simulink model "backups"  (R2024a)
settings: Solver=VariableStepAuto  StartTime=0.0  StopTime=10.0  RelTol=1e-3
values from neighbouring files (symbols this model uses):
  AttKd_x = inp(4,2).Var2    [SFF_Simulator_Entradas.m]
  AttKd_y = inp(5,2).Var2    [SFF_Simulator_Entradas.m]
  AttKd_z = inp(6,2).Var2    [SFF_Simulator_Entradas.m]
  AttKp_x = inp(1,2).Var2    [SFF_Simulator_Entradas.m]
  AttKp_y = inp(2,2).Var2    [SFF_Simulator_Entradas.m]
  AttKp_z = inp(3,2).Var2    [SFF_Simulator_Entradas.m]
  B = inp(8,2).Var2    [SFF_Simulator_Entradas.m]
  beta = inp(2,2).Var2    [SFF_Simulator_Entradas.m]
  Cd1 = inp(4,2).Var2    [SFF_Simulator_Entradas.m]
  cdgps = inp(1,2).Var2    [SFF_Simulator_Entradas.m]
  estrelas = inp(4,2).Var2    [SFF_Simulator_Entradas.m]
  estrelas_bias = inp(6,2).Var2    [SFF_Simulator_Entradas.m]
  estrelas_ruido = inp(5,2).Var2    [SFF_Simulator_Entradas.m]
  Fn = inp(2,2).Var2    [SFF_Simulator_Entradas.m]
  gps_bias = inp(3,2).Var2    [SFF_Simulator_Entradas.m]
  gps_ruido = inp(2,2).Var2    [SFF_Simulator_Entradas.m]
  Iw = inp(7,2).Var2    [SFF_Simulator_Entradas.m]
  Ixx = inp(7,2).Var2    [SFF_Simulator_Entradas.m]
  Iyy = inp(8,2).Var2    [SFF_Simulator_Entradas.m]
  Izz = inp(9,2).Var2    [SFF_Simulator_Entradas.m]
  Km = inp(3,2).Var2    [SFF_Simulator_Entradas.m]
  Kv = inp(9,2).Var2    [SFF_Simulator_Entradas.m]
  L1 = inp(5,2).Var2    [SFF_Simulator_Entradas.m]
  limCorrente = inp(4,2).Var2    [SFF_Simulator_Entradas.m]
  limVolt = inp(5,2).Var2    [SFF_Simulator_Entradas.m]
  m1 = inp(6,2).Var2    [SFF_Simulator_Entradas.m]
  magne = inp(10,2).Var2    [SFF_Simulator_Entradas.m]
  magne_bias = inp(12,2).Var2    [SFF_Simulator_Entradas.m]
  magne_ruido = inp(11,2).Var2    [SFF_Simulator_Entradas.m]
  man = inp(1,2).Var2    [SFF_Simulator_Entradas.m]
  OrbKd_x = inp(3,2).Var2    [SFF_Simulator_Entradas.m]
  OrbKd_y = inp(6,2).Var2    [SFF_Simulator_Entradas.m]
  OrbKd_z = inp(9,2).Var2    [SFF_Simulator_Entradas.m]
  OrbKi_x = inp(2,2).Var2    [SFF_Simulator_Entradas.m]
  OrbKi_y = inp(5,2).Var2    [SFF_Simulator_Entradas.m]
  OrbKi_z = inp(8,2).Var2    [SFF_Simulator_Entradas.m]
  OrbKp_x = inp(1,2).Var2    [SFF_Simulator_Entradas.m]
  OrbKp_y = inp(4,2).Var2    [SFF_Simulator_Entradas.m]
  OrbKp_z = inp(7,2).Var2    [SFF_Simulator_Entradas.m]
  propForcaAtivo = inp(1,2).Var2    [SFF_Simulator_Entradas.m]
  Rm = inp(6,2).Var2    [SFF_Simulator_Entradas.m]
  rodaAtivo = inp(1,2).Var2    [SFF_Simulator_Entradas.m]
  RodKi = inp(1,2).Var2    [SFF_Simulator_Entradas.m]
  sat_torquerod = inp(14,2).Var2    [SFF_Simulator_Entradas.m]
  torqrodAtivo = inp(1,2).Var2    [SFF_Simulator_Entradas.m]
undefined symbols (not defined in the file or in its folder): IAU, J2, mi, omega_E, propMomentoAtivo, Re, sat_rodareacao, WMM2020
libraries: dspsrcs4 x19, aerolibtransform2 x2, aerolibgravity2 x2, simulink x1
(part 2 of 4)

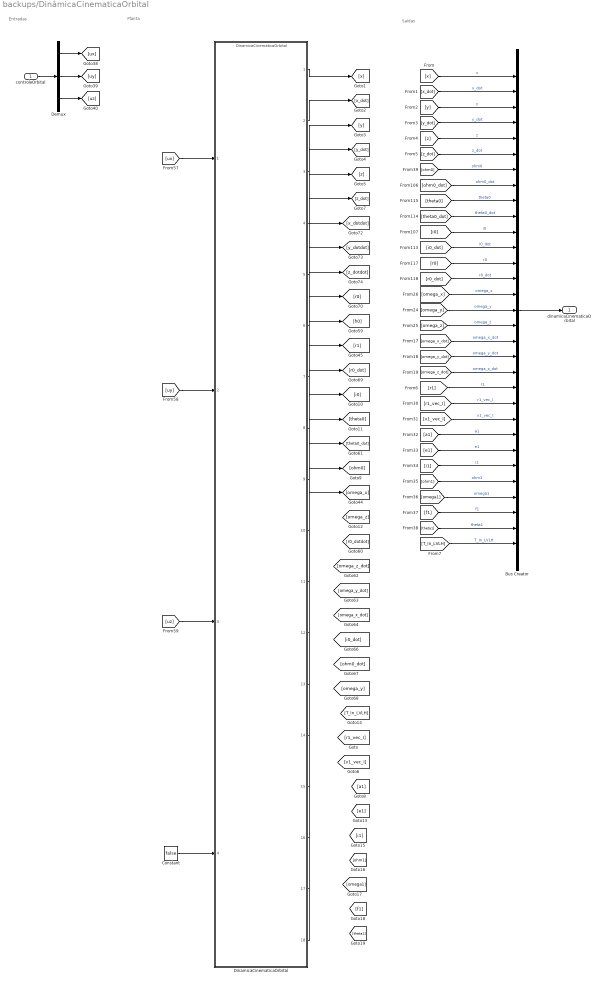
== system backups/DinâmicaCinematicaOrbital ==
  note: Entradas
  note: Saídas
  note: Planta
  controleOrbital : Inport  OutDataTypeStr=double
  Bus Creator : BusCreator  Inputs=31
  Constant : Constant  Value=false
  Demux : Demux  Outputs=3
  DinamicaCinematicaOrbital : ModelReference  ModelNameDialog=DinamicaCinematicaOrbital  ModelReferenceVersion=5.18
  dinamicaCinematicaOrbital : Outport
  wires:
  [x] -> Bus Creator/1  "x"
  [z_dot] -> Bus Creator/6  "z_dot"
  [y] -> Bus Creator/3  "y"
  [z] -> Bus Creator/5  "z"
  [x_dot] -> Bus Creator/2  "x_dot"
  [y_dot] -> Bus Creator/4  "y_dot"
  Bus Creator/1 -> dinamicaCinematicaOrbital/1
  controleOrbital/1 -> Demux/1
  Demux/1 -> [ux]
  Demux/2 -> [uy]
  Demux/3 -> [uz]
  [ohm0] -> Bus Creator/7  "ohm0"
  [ohm0_dot] -> Bus Creator/8  "ohm0_dot"
  [theta0] -> Bus Creator/9  "theta0"
  [theta0_dot] -> Bus Creator/10  "theta0_dot"
  [i0] -> Bus Creator/11  "i0"
  [i0_dot] -> Bus Creator/12  "i0_dot"
  [r0] -> Bus Creator/13  "r0"
  [r0_dot] -> Bus Creator/14  "r0_dot"
  [omega_x] -> Bus Creator/15  "omega_x"
  [omega_y] -> Bus Creator/16  "omega_y"
  [omega_z] -> Bus Creator/17  "omega_z"
  [omega_x_dot] -> Bus Creator/18  "omega_x_dot"
  [omega_y_dot] -> Bus Creator/19  "omega_y_dot"
  [omega_z_dot] -> Bus Creator/20  "omega_z_dot"
  [r1] -> Bus Creator/21  "r1"
  [r1_vec_I] -> Bus Creator/22  "r1_vec_I"
  [v1_vec_I] -> Bus Creator/23  "v1_vec_I"
  [a1] -> Bus Creator/24  "a1"
  [e1] -> Bus Creator/25  "e1"
  [i1] -> Bus Creator/26  "i1"
  [ohm1] -> Bus Creator/27  "ohm1"
  [omega1] -> Bus Creator/28  "omega1"
  [f1] -> Bus Creator/29  "f1"
  [theta1] -> Bus Creator/30  "theta1"
  [T_In_LVLH] -> Bus Creator/31  "T_In_LVLH"
  [ux] -> DinamicaCinematicaOrbital/1
  [uy] -> DinamicaCinematicaOrbital/2
  [uz] -> DinamicaCinematicaOrbital/3
  Constant/1 -> DinamicaCinematicaOrbital/4
  DinamicaCinematicaOrbital/7 -> [x_dotdot]
  DinamicaCinematicaOrbital/8 -> [y_dotdot]
  DinamicaCinematicaOrbital/9 -> [z_dotdot]
  DinamicaCinematicaOrbital/10 -> [r0]
  DinamicaCinematicaOrbital/11 -> [h0]
  DinamicaCinematicaOrbital/12 -> [r1]
  DinamicaCinematicaOrbital/13 -> [r0_dot]
  DinamicaCinematicaOrbital/14 -> [i0]
  DinamicaCinematicaOrbital/15 -> [theta0]
  DinamicaCinematicaOrbital/16 -> [theta0_dot]
  DinamicaCinematicaOrbital/17 -> [ohm0]
  DinamicaCinematicaOrbital/18 -> [omega_x]
  ? -> [omega_z]
  ? -> [r0_dotdot]
  ? -> [omega_z_dot]
  ? -> [omega_y_dot]
  ? -> [omega_x_dot]
  ? -> [i0_dot]
  ? -> [ohm0_dot]
  ? -> [omega_y]
  ? -> [T_In_LVLH]
  DinamicaCinematicaOrbital/1 -> [x]
  DinamicaCinematicaOrbital/2 -> [x_dot]
  DinamicaCinematicaOrbital/4 -> [y_dot]
  DinamicaCinematicaOrbital/5 -> [z]
  DinamicaCinematicaOrbital/6 -> [z_dot]
  DinamicaCinematicaOrbital/3 -> [y]
  ? -> [r1_vec_I]
  ? -> [v1_vec_I]
  ? -> [theta1]
  ? -> [f1]
  ? -> [omega1]
  ? -> [ohm1]
  ? -> [i1]
  ? -> [e1]
  ? -> [a1]

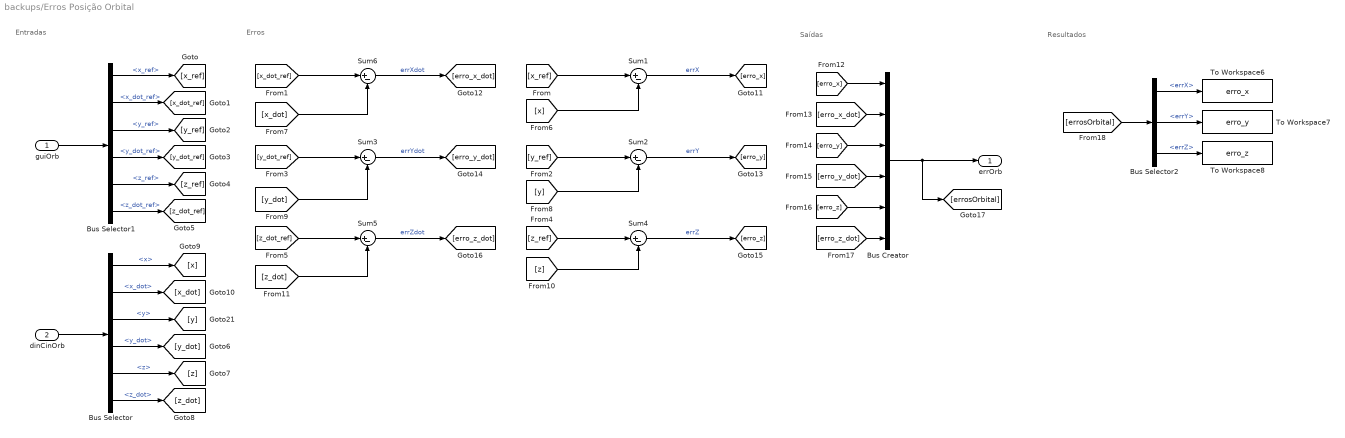
== system backups/Erros Posição Orbital ==
  note: Saídas
  note: Erros
  note: Entradas
  note: Resultados
  guiOrb : Inport
  dinCinOrb : Inport  Port=2
  Bus Creator : BusCreator  Inputs=6
  Bus Selector : BusSelector  OutputSignals=x,x_dot,y,y_dot,z,z_dot
  Bus Selector1 : BusSelector  OutputSignals=x_ref,x_dot_ref,y_ref,y_dot_ref,z_ref,z_dot_ref
  Bus Selector2 : BusSelector  OutputSignals=errX,errY,errZ
  Sum{1..6} (6 alike) : Sum  Inputs=|+-
  To Workspace6 : ToWorkspace  VariableName=erro_x  SampleTime=-1
      settings: Save2DSignal=2-D array (concatenate along first dimension)
  To Workspace7 : ToWorkspace  VariableName=erro_y  SampleTime=-1
      settings: Save2DSignal=2-D array (concatenate along first dimension)
  To Workspace8 : ToWorkspace  VariableName=erro_z  SampleTime=-1
      settings: Save2DSignal=2-D array (concatenate along first dimension)
  errOrb : Outport
  wires:
  [x] -> Sum1/2
  [x_dot] -> Sum6/2
  [x_dot_ref] -> Sum6/1
  [x_ref] -> Sum1/1
  Sum6/1 -> [erro_x_dot]  "errXdot"
  Sum1/1 -> [erro_x]  "errX"
  Sum3/1 -> [erro_y_dot]  "errYdot"
  Sum2/1 -> [erro_y]  "errY"
  [y] -> Sum2/2
  [y_dot] -> Sum3/2
  [y_ref] -> Sum2/1
  [y_dot_ref] -> Sum3/1
  Sum5/1 -> [erro_z_dot]  "errZdot"
  Sum4/1 -> [erro_z]  "errZ"
  [z_dot] -> Sum5/2
  [z_dot_ref] -> Sum5/1
  [z] -> Sum4/2
  [z_ref] -> Sum4/1
  Bus Selector1/4 -> [y_dot_ref]  "<y_dot_ref>"
  Bus Selector1/2 -> [x_dot_ref]  "<x_dot_ref>"
  guiOrb/1 -> Bus Selector1/1
  Bus Selector1/6 -> [z_dot_ref]  "<z_dot_ref>"
  Bus Selector1/3 -> [y_ref]  "<y_ref>"
  Bus Selector1/1 -> [x_ref]  "<x_ref>"
  Bus Selector1/5 -> [z_ref]  "<z_ref>"
  Bus Selector/1 -> [x]  "<x>"
  Bus Selector/4 -> [y_dot]  "<y_dot>"
  Bus Selector/3 -> [y]  "<y>"
  Bus Selector/6 -> [z_dot]  "<z_dot>"
  Bus Selector/5 -> [z]  "<z>"
  Bus Selector/2 -> [x_dot]  "<x_dot>"
  dinCinOrb/1 -> Bus Selector/1
  [erro_x] -> Bus Creator/1
  [erro_x_dot] -> Bus Creator/2
  [erro_y] -> Bus Creator/3
  [erro_y_dot] -> Bus Creator/4
  [erro_z] -> Bus Creator/5
  [erro_z_dot] -> Bus Creator/6
  Bus Selector2/2 -> To Workspace7/1  "<errY>"
  Bus Selector2/3 -> To Workspace8/1  "<errZ>"
  Bus Selector2/1 -> To Workspace6/1  "<errX>"
  [errosOrbital] -> Bus Selector2/1
  Bus Creator/1 -> [errosOrbital], errOrb/1

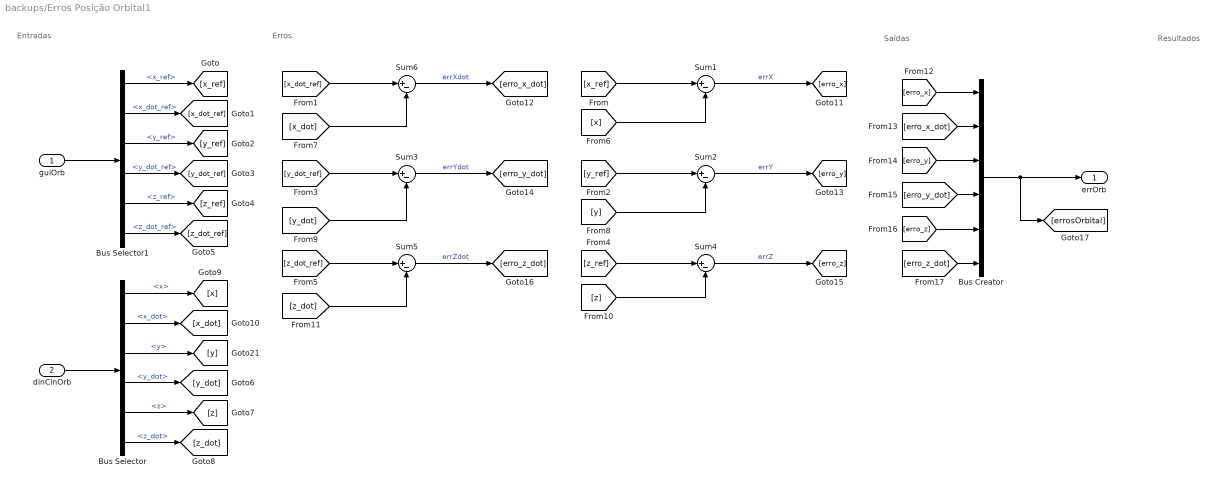
== system backups/Erros Posição Orbital1 ==
  note: Saídas
  note: Erros
  note: Entradas
  note: Resultados
  guiOrb : Inport
  dinCinOrb : Inport  Port=2
  Bus Creator : BusCreator  Inputs=6
  Bus Selector : BusSelector  OutputSignals=x,x_dot,y,y_dot,z,z_dot
  Bus Selector1 : BusSelector  OutputSignals=x_ref,x_dot_ref,y_ref,y_dot_ref,z_ref,z_dot_ref
  Sum{1..6} (6 alike) : Sum  Inputs=|+-
  errOrb : Outport
  wires:
  [x] -> Sum1/2
  [x_dot] -> Sum6/2
  [x_dot_ref] -> Sum6/1
  [x_ref] -> Sum1/1
  Sum6/1 -> [erro_x_dot]  "errXdot"
  Sum1/1 -> [erro_x]  "errX"
  Sum3/1 -> [erro_y_dot]  "errYdot"
  Sum2/1 -> [erro_y]  "errY"
  [y] -> Sum2/2
  [y_dot] -> Sum3/2
  [y_ref] -> Sum2/1
  [y_dot_ref] -> Sum3/1
  Sum5/1 -> [erro_z_dot]  "errZdot"
  Sum4/1 -> [erro_z]  "errZ"
  [z_dot] -> Sum5/2
  [z_dot_ref] -> Sum5/1
  [z] -> Sum4/2
  [z_ref] -> Sum4/1
  Bus Selector1/4 -> [y_dot_ref]  "<y_dot_ref>"
  Bus Selector1/2 -> [x_dot_ref]  "<x_dot_ref>"
  guiOrb/1 -> Bus Selector1/1
  Bus Selector1/6 -> [z_dot_ref]  "<z_dot_ref>"
  Bus Selector1/3 -> [y_ref]  "<y_ref>"
  Bus Selector1/1 -> [x_ref]  "<x_ref>"
  Bus Selector1/5 -> [z_ref]  "<z_ref>"
  Bus Selector/1 -> [x]  "<x>"
  Bus Selector/4 -> [y_dot]  "<y_dot>"
  Bus Selector/3 -> [y]  "<y>"
  Bus Selector/6 -> [z_dot]  "<z_dot>"
  Bus Selector/5 -> [z]  "<z>"
  Bus Selector/2 -> [x_dot]  "<x_dot>"
  dinCinOrb/1 -> Bus Selector/1
  [erro_x] -> Bus Creator/1
  [erro_x_dot] -> Bus Creator/2
  [erro_y] -> Bus Creator/3
  [erro_y_dot] -> Bus Creator/4
  [erro_z] -> Bus Creator/5
  [erro_z_dot] -> Bus Creator/6
  Bus Creator/1 -> [errosOrbital], errOrb/1

== system backups/Erros Quatérnions ==
  note: Erros
  note: Saídas
  note: Entradas
  q_ref : Inport
  q_rel : Inport  Port=2
  MATLAB Function4 : MATLAB Function  TreatAsAtomicUnit=on
  q_erro : Outport
  wires:
  [q_ref] -> MATLAB Function4/1(q_d)
  [q_rel] -> MATLAB Function4/2(q)
  MATLAB Function4/1(q_error) -> [q_erro]  "q_erro"
  [q_erro] -> q_erro/1
  q_rel/1 -> [q_rel]
  q_ref/1 -> [q_ref]

== system backups/Erros Quatérnions1 ==
  note: Erros
  note: Saídas
  note: Entradas
  q_ref : Inport
  q_rel : Inport  Port=2
  MATLAB Function4 : MATLAB Function  TreatAsAtomicUnit=on
  Scope : Scope
  q_erro : Outport
  wires:
  [q_ref] -> MATLAB Function4/1(q_d)
  [q_rel] -> MATLAB Function4/2(q)
  MATLAB Function4/1(q_error) -> [q_erro]  "q_erro"
  [q_erro] -> Scope/1, q_erro/1
  q_rel/1 -> [q_rel]
  q_ref/1 -> [q_ref]

== system backups/Guiamento Atitude ==
  note: Entradas
  note: Guiamento de Atitude
  note: Saídas
  note: Resultados
  dinCinOrb : Inport
  Bus Selector1 : BusSelector  OutputSignals=T_In_LVLH,r0,ohm1,i1,theta1,r1_vec_I
  "Euler -> Quatérnions" : MATLAB Function  TreatAsAtomicUnit=on
  GuiamentoAtitude : ModelReference  ModelNameDialog=GuiamentoAtitude  ModelReferenceVersion=3.9
  To Workspace12 : ToWorkspace  VariableName=phi_ref  SampleTime=-1
      settings: Save2DSignal=2-D array (concatenate along first dimension)
  To Workspace13 : ToWorkspace  VariableName=theta_ref  SampleTime=-1
      settings: Save2DSignal=2-D array (concatenate along first dimension)
  To Workspace14 : ToWorkspace  VariableName=psi_ref  SampleTime=-1
      settings: Save2DSignal=2-D array (concatenate along first dimension)
  q_ref : Outport
  wires:
  dinCinOrb/1 -> Bus Selector1/1
  GuiamentoAtitude/2 -> [theta_ref]
  [r0] -> GuiamentoAtitude/2
  [ohm1] -> GuiamentoAtitude/3
  [theta1] -> GuiamentoAtitude/5
  GuiamentoAtitude/1 -> [phi_ref]
  GuiamentoAtitude/3 -> [psi_ref]
  [r1_vec_I] -> GuiamentoAtitude/6
  [i1] -> GuiamentoAtitude/4
  [T_In_LVLH] -> GuiamentoAtitude/1
  [theta_ref] -> To Workspace13/1
  [phi_ref] -> To Workspace12/1
  [phi_ref] -> "Euler -> Quatérnions"/1(phi_ref)
  [psi_ref] -> "Euler -> Quatérnions"/3(psi_ref)
  [psi_ref] -> To Workspace14/1
  [theta_ref] -> "Euler -> Quatérnions"/2(theta_ref)
  "Euler -> Quatérnions"/1(q_ref) -> q_ref/1
  Bus Selector1/3 -> [ohm1]  "<ohm1>"
  Bus Selector1/5 -> [theta1]  "<theta1>"
  Bus Selector1/2 -> [r0]  "<r0>"
  Bus Selector1/4 -> [i1]  "<i1>"
  Bus Selector1/1 -> [T_In_LVLH]  "<T_In_LVLH>"
  Bus Selector1/6 -> [r1_vec_I]  "<r1_vec_I>"

== system backups/Guiamento Atitude1 ==
  note: Entradas
  note: Guiamento de Atitude
  note: Saídas
  note: Resultados
  dinCinOrb : Inport
  Bus Selector1 : BusSelector  OutputSignals=T_In_LVLH,r0,ohm1,i1,theta1,r1_vec_I
  "Euler -> Quatérnions" : MATLAB Function  TreatAsAtomicUnit=on
  GuiamentoAtitude : ModelReference  ModelNameDialog=GuiamentoAtitude  ModelReferenceVersion=3.9
  To Workspace12 : ToWorkspace  VariableName=phi_ref  SampleTime=-1
      settings: Save2DSignal=2-D array (concatenate along first dimension)
  To Workspace13 : ToWorkspace  VariableName=theta_ref  SampleTime=-1
      settings: Save2DSignal=2-D array (concatenate along first dimension)
  To Workspace14 : ToWorkspace  VariableName=psi_ref  SampleTime=-1
      settings: Save2DSignal=2-D array (concatenate along first dimension)
  q_ref : Outport
  wires:
  dinCinOrb/1 -> Bus Selector1/1
  GuiamentoAtitude/2 -> [theta_ref]
  [r0] -> GuiamentoAtitude/2
  [ohm1] -> GuiamentoAtitude/3
  [theta1] -> GuiamentoAtitude/5
  GuiamentoAtitude/1 -> [phi_ref]
  GuiamentoAtitude/3 -> [psi_ref]
  [r1_vec_I] -> GuiamentoAtitude/6
  [i1] -> GuiamentoAtitude/4
  [T_In_LVLH] -> GuiamentoAtitude/1
  [theta_ref] -> To Workspace13/1
  [phi_ref] -> To Workspace12/1
  [phi_ref] -> "Euler -> Quatérnions"/1(phi_ref)
  [psi_ref] -> "Euler -> Quatérnions"/3(psi_ref)
  [psi_ref] -> To Workspace14/1
  [theta_ref] -> "Euler -> Quatérnions"/2(theta_ref)
  "Euler -> Quatérnions"/1(q_ref) -> q_ref/1
  Bus Selector1/3 -> [ohm1]  "<ohm1>"
  Bus Selector1/5 -> [theta1]  "<theta1>"
  Bus Selector1/2 -> [r0]  "<r0>"
  Bus Selector1/4 -> [i1]  "<i1>"
  Bus Selector1/1 -> [T_In_LVLH]  "<T_In_LVLH>"
  Bus Selector1/6 -> [r1_vec_I]  "<r1_vec_I>"

== system backups/Guiamento Orbital ==
  note: Saídas
  note: Guiamento Orbital
  note: Resultados
  Bus Creator : BusCreator  Inputs=12
  Bus Selector : BusSelector  OutputSignals=x_ref,y_ref,z_ref
  Constant13 : Constant  Value=man  OutDataTypeStr=boolean
  DinamicaCinematicaOrbital : ModelReference  ModelNameDialog=DinamicaCinematicaOrbital  ModelReferenceVersion=5.18
  Terminator{,1..5} (6 alike) : Terminator
  To Workspace : ToWorkspace  VariableName=x_ref  SampleTime=-1
      settings: Save2DSignal=2-D array (concatenate along first dimension)
  To Workspace1 : ToWorkspace  VariableName=y_ref  SampleTime=-1
      settings: Save2DSignal=2-D array (concatenate along first dimension)
  To Workspace2 : ToWorkspace  VariableName=z_ref  SampleTime=-1
      settings: Save2DSignal=2-D array (concatenate along first dimension)
  ux : Constant  Value=0
  uy : Constant  Value=0
  uz : Constant  Value=0
  guiOrb : Outport
  wires:
  [x] -> Bus Creator/1  "x_ref"
  [x_dot] -> Bus Creator/2  "x_dot_ref"
  [y] -> Bus Creator/3  "y_ref"
  [y_dot] -> Bus Creator/4  "y_dot_ref"
  [z] -> Bus Creator/5  "z_ref"
  [z_dot] -> Bus Creator/6  "z_dot_ref"
  Bus Creator/1 -> [guiOrb], guiOrb/1
  ux/1 -> DinamicaCinematicaOrbital/1
  uy/1 -> DinamicaCinematicaOrbital/2
  uz/1 -> DinamicaCinematicaOrbital/3
  Constant13/1 -> DinamicaCinematicaOrbital/4
  [r0] -> Bus Creator/8  "r0"
  [T_In_LVLH] -> Bus Creator/7  "T_In_LVLH"
  [ohm1] -> Bus Creator/9  "ohm1"
  [i1] -> Bus Creator/10  "i1"
  [theta1] -> Bus Creator/11  "theta1"
  [r1_vec_I] -> Bus Creator/12  "r1_vec_I"
  Bus Selector/3 -> To Workspace2/1  "<z_ref>"
  Bus Selector/2 -> To Workspace1/1  "<y_ref>"
  Bus Selector/1 -> To Workspace/1  "<x_ref>"
  [guiOrb] -> Bus Selector/1
  DinamicaCinematicaOrbital/1 -> [x]
  DinamicaCinematicaOrbital/2 -> [x_dot]
  DinamicaCinematicaOrbital/3 -> [y]
  DinamicaCinematicaOrbital/4 -> [y_dot]
  DinamicaCinematicaOrbital/5 -> [z]
  DinamicaCinematicaOrbital/6 -> [z_dot]
  DinamicaCinematicaOrbital/7 -> [r0]
  DinamicaCinematicaOrbital/8 -> Terminator/1
  DinamicaCinematicaOrbital/9 -> Terminator1/1
  DinamicaCinematicaOrbital/10 -> Terminator2/1
  DinamicaCinematicaOrbital/11 -> Terminator4/1
  DinamicaCinematicaOrbital/12 -> Terminator5/1
  DinamicaCinematicaOrbital/18 -> [theta1]
  DinamicaCinematicaOrbital/17 -> [ohm1]
  DinamicaCinematicaOrbital/16 -> [i1]
  DinamicaCinematicaOrbital/15 -> [r1_vec_I]
  DinamicaCinematicaOrbital/14 -> [T_In_LVLH]
  DinamicaCinematicaOrbital/13 -> Terminator3/1

== system backups/Guiamento Orbital1 ==
  note: Saídas
  note: Guiamento Orbital
  note: Resultados
  Bus Creator : BusCreator  Inputs=12
  Bus Selector : BusSelector  OutputSignals=x_ref,y_ref,z_ref
  Constant13 : Constant  Value=man  OutDataTypeStr=boolean
  DinamicaCinematicaOrbital : ModelReference  ModelNameDialog=DinamicaCinematicaOrbital  ModelReferenceVersion=5.18
  Terminator{,1..5} (6 alike) : Terminator
  To Workspace : ToWorkspace  VariableName=x_ref  SampleTime=-1
      settings: Save2DSignal=2-D array (concatenate along first dimension)
  To Workspace1 : ToWorkspace  VariableName=y_ref  SampleTime=-1
      settings: Save2DSignal=2-D array (concatenate along first dimension)
  To Workspace2 : ToWorkspace  VariableName=z_ref  SampleTime=-1
      settings: Save2DSignal=2-D array (concatenate along first dimension)
  ux : Constant  Value=0
  uy : Constant  Value=0
  uz : Constant  Value=0
  guiOrb : Outport
  wires:
  [x] -> Bus Creator/1  "x_ref"
  [x_dot] -> Bus Creator/2  "x_dot_ref"
  [y] -> Bus Creator/3  "y_ref"
  [y_dot] -> Bus Creator/4  "y_dot_ref"
  [z] -> Bus Creator/5  "z_ref"
  [z_dot] -> Bus Creator/6  "z_dot_ref"
  Bus Creator/1 -> [guiOrb], guiOrb/1
  ux/1 -> DinamicaCinematicaOrbital/1
  uy/1 -> DinamicaCinematicaOrbital/2
  uz/1 -> DinamicaCinematicaOrbital/3
  Constant13/1 -> DinamicaCinematicaOrbital/4
  [r0] -> Bus Creator/8  "r0"
  [T_In_LVLH] -> Bus Creator/7  "T_In_LVLH"
  [ohm1] -> Bus Creator/9  "ohm1"
  [i1] -> Bus Creator/10  "i1"
  [theta1] -> Bus Creator/11  "theta1"
  [r1_vec_I] -> Bus Creator/12  "r1_vec_I"
  Bus Selector/3 -> To Workspace2/1  "<z_ref>"
  Bus Selector/2 -> To Workspace1/1  "<y_ref>"
  Bus Selector/1 -> To Workspace/1  "<x_ref>"
  [guiOrb] -> Bus Selector/1
  DinamicaCinematicaOrbital/1 -> [x]
  DinamicaCinematicaOrbital/2 -> [x_dot]
  DinamicaCinematicaOrbital/3 -> [y]
  DinamicaCinematicaOrbital/4 -> [y_dot]
  DinamicaCinematicaOrbital/5 -> [z]
  DinamicaCinematicaOrbital/6 -> [z_dot]
  DinamicaCinematicaOrbital/7 -> [r0]
  DinamicaCinematicaOrbital/8 -> Terminator/1
  DinamicaCinematicaOrbital/9 -> Terminator1/1
  DinamicaCinematicaOrbital/10 -> Terminator2/1
  DinamicaCinematicaOrbital/11 -> Terminator4/1
  DinamicaCinematicaOrbital/12 -> Terminator5/1
  DinamicaCinematicaOrbital/18 -> [theta1]
  DinamicaCinematicaOrbital/17 -> [ohm1]
  DinamicaCinematicaOrbital/16 -> [i1]
  DinamicaCinematicaOrbital/15 -> [r1_vec_I]
  DinamicaCinematicaOrbital/14 -> [T_In_LVLH]
  DinamicaCinematicaOrbital/13 -> Terminator3/1

== system backups/GuiamentoAtitude ==
  note: Entradas
  note: Planta
  note: Saídas
  dinamicaCinematicaOrbital : Inport
  Bus Creator : BusCreator  Inputs=3
  Bus Selector : BusSelector  OutputSignals=T_In_LVLH,r0,ohm1,i1,theta1,r1_vec_I
  "Euler -> Quatérnions" : MATLAB Function  TreatAsAtomicUnit=on
  GuiamentoAtitude1 : ModelReference  ModelNameDialog=GuiamentoAtitude  ModelReferenceVersion=3.9
  eulerRef : Outport
  q_ref : Outport  Port=2
  wires:
  dinamicaCinematicaOrbital/1 -> Bus Selector/1
  Bus Selector/1 -> [T_In_LVLH]  "<T_In_LVLH>"
  Bus Selector/2 -> [r0]  "<r0>"
  Bus Selector/3 -> [ohm1]  "<ohm1>"
  Bus Selector/4 -> [i1]  "<i1>"
  Bus Selector/5 -> [theta1]  "<theta1>"
  Bus Selector/6 -> [r1_vec_I]  "<r1_vec_I>"
  GuiamentoAtitude1/2 -> [theta_ref]
  [r0] -> GuiamentoAtitude1/2
  [ohm1] -> GuiamentoAtitude1/3
  [theta1] -> GuiamentoAtitude1/5
  GuiamentoAtitude1/1 -> [phi_ref]
  GuiamentoAtitude1/3 -> [psi_ref]
  [r1_vec_I] -> GuiamentoAtitude1/6
  [i1] -> GuiamentoAtitude1/4
  [T_In_LVLH] -> GuiamentoAtitude1/1
  Bus Creator/1 -> eulerRef/1
  [theta_ref] -> Bus Creator/2  "theta_ref"
  [phi_ref] -> Bus Creator/1  "phi_ref"
  [phi_ref] -> "Euler -> Quatérnions"/1(phi_ref)
  [psi_ref] -> "Euler -> Quatérnions"/3(psi_ref)
  [psi_ref] -> Bus Creator/3  "psi_ref"
  [theta_ref] -> "Euler -> Quatérnions"/2(theta_ref)
  "Euler -> Quatérnions"/1(q_ref) -> q_ref/1

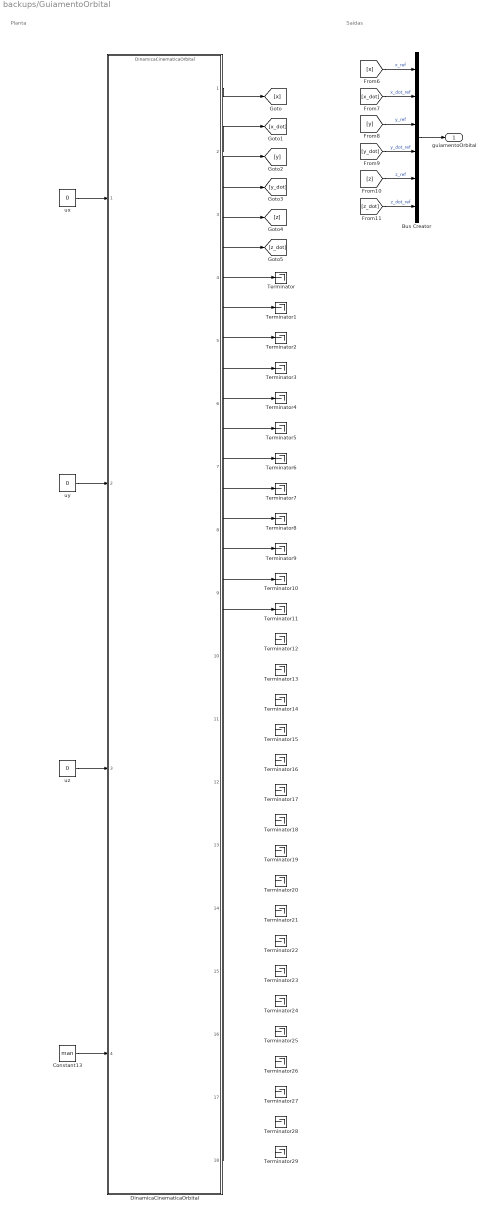
== system backups/GuiamentoOrbital ==
  note: Saídas
  note: Planta
  Bus Creator : BusCreator  Inputs=6
  Constant13 : Constant  Value=man  OutDataTypeStr=boolean
  DinamicaCinematicaOrbital : ModelReference  ModelNameDialog=DinamicaCinematicaOrbital  ModelReferenceVersion=5.18
  Terminator{,1..29} (30 alike) : Terminator
  ux : Constant  Value=0
  uy : Constant  Value=0
  uz : Constant  Value=0
  guiamentoOrbital : Outport
  wires:
  [x] -> Bus Creator/1  "x_ref"
  [x_dot] -> Bus Creator/2  "x_dot_ref"
  [y] -> Bus Creator/3  "y_ref"
  [y_dot] -> Bus Creator/4  "y_dot_ref"
  [z] -> Bus Creator/5  "z_ref"
  [z_dot] -> Bus Creator/6  "z_dot_ref"
  Bus Creator/1 -> guiamentoOrbital/1
  ux/1 -> DinamicaCinematicaOrbital/1
  uy/1 -> DinamicaCinematicaOrbital/2
  uz/1 -> DinamicaCinematicaOrbital/3
  DinamicaCinematicaOrbital/1 -> [x]
  DinamicaCinematicaOrbital/2 -> [x_dot]
  DinamicaCinematicaOrbital/3 -> [y]
  DinamicaCinematicaOrbital/4 -> [y_dot]
  DinamicaCinematicaOrbital/5 -> [z]
  DinamicaCinematicaOrbital/6 -> [z_dot]
  DinamicaCinematicaOrbital/7 -> Terminator/1
  DinamicaCinematicaOrbital/8 -> Terminator1/1
  DinamicaCinematicaOrbital/9 -> Terminator2/1
  DinamicaCinematicaOrbital/10 -> Terminator3/1
  DinamicaCinematicaOrbital/11 -> Terminator4/1
  DinamicaCinematicaOrbital/12 -> Terminator5/1
  DinamicaCinematicaOrbital/13 -> Terminator6/1
  DinamicaCinematicaOrbital/14 -> Terminator7/1
  DinamicaCinematicaOrbital/15 -> Terminator8/1
  DinamicaCinematicaOrbital/16 -> Terminator9/1
  DinamicaCinematicaOrbital/17 -> Terminator10/1
  DinamicaCinematicaOrbital/18 -> Terminator11/1
  ? -> Terminator12/1
  ? -> Terminator13/1
  ? -> Terminator14/1
  ? -> Terminator15/1
  ? -> Terminator16/1
  ? -> Terminator17/1
  ? -> Terminator18/1
  ? -> Terminator19/1
  Constant13/1 -> DinamicaCinematicaOrbital/4
  ? -> Terminator20/1
  ? -> Terminator21/1
  ? -> Terminator22/1
  ? -> Terminator23/1
  ? -> Terminator24/1
  ? -> Terminator25/1
  ? -> Terminator26/1
  ? -> Terminator27/1
  ? -> Terminator28/1
  ? -> Terminator29/1

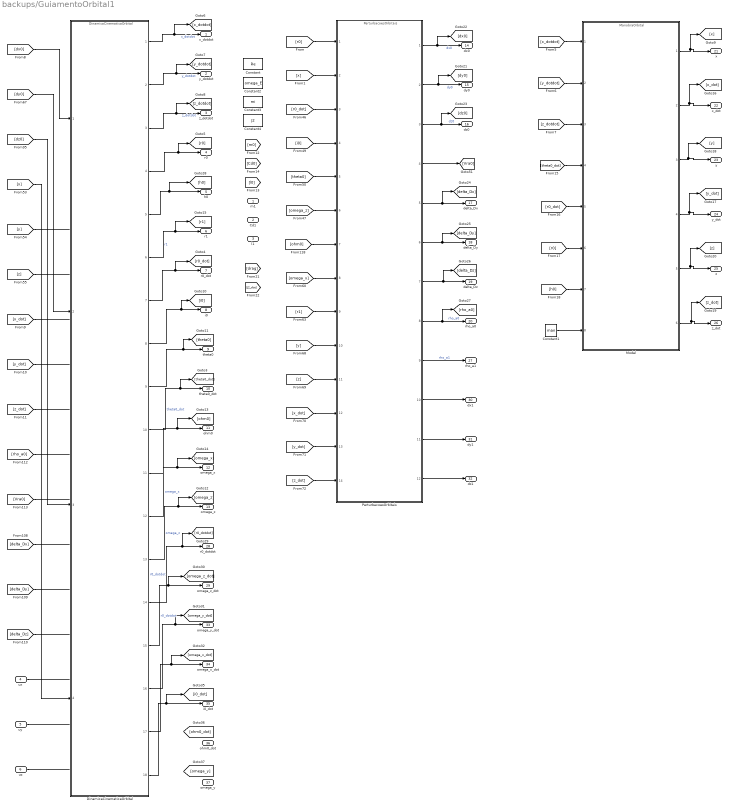
== system backups/GuiamentoOrbital1 ==
  m1 : Inport  OutDataTypeStr=double  PortDimensions=1
  Cd1 : Inport  Port=2  OutDataTypeStr=double  PortDimensions=1
  l1 : Inport  Port=3  OutDataTypeStr=double  PortDimensions=1
  ux : Inport  Port=4  OutDataTypeStr=double  PortDimensions=1
  uy : Inport  Port=5  OutDataTypeStr=double  PortDimensions=1
  uz : Inport  Port=6  OutDataTypeStr=double  PortDimensions=1
  Constant : Constant  Value=Re
  Constant1 : Constant  Value=man
  Constant2 : Constant  Value=omega_E
  Constant3 : Constant  Value=mi
  Constant4 : Constant  Value=J2
  DinamicaCinematicaOrbital : ModelReference  ModelNameDialog=DinamicaCinematicaOrbital  ModelReferenceVersion=5.18
  Model : ModelReference  ModelNameDialog=ManobraOrbital.slx  ModelReferenceVersion=4.15
  PerturbacoesOrbitais : ModelReference  ModelNameDialog=PerturbacoesOrbitais  ModelReferenceVersion=4.1
  x_dotdot : Outport  OutDataTypeStr=double  PortDimensions=1  SampleTime=0
  y_dotdot : Outport  Port=2  OutDataTypeStr=double  PortDimensions=1  SampleTime=0
  z_dotdot : Outport  Port=3  OutDataTypeStr=double  PortDimensions=1  SampleTime=0
  r0 : Outport  Port=4  OutDataTypeStr=double  PortDimensions=1  SampleTime=0
  h0 : Outport  Port=5  OutDataTypeStr=double  PortDimensions=1  SampleTime=0
  r1 : Outport  Port=6  OutDataTypeStr=double  PortDimensions=1  SampleTime=0
  r0_dot : Outport  Port=7  OutDataTypeStr=double  PortDimensions=1  SampleTime=0
  i0 : Outport  Port=8  OutDataTypeStr=double  PortDimensions=1  SampleTime=0
  theta0 : Outport  Port=9  OutDataTypeStr=double  PortDimensions=1  SampleTime=0
  theta0_dot : Outport  Port=10  OutDataTypeStr=double  PortDimensions=1  SampleTime=0
  ohm0 : Outport  Port=11  OutDataTypeStr=double  PortDimensions=1  SampleTime=0
  omega_x : Outport  Port=12  OutDataTypeStr=double  PortDimensions=1  SampleTime=0
  omega_z : Outport  Port=13  OutDataTypeStr=double  PortDimensions=1  SampleTime=0
  dx0 : Outport  Port=14  OutDataTypeStr=double  PortDimensions=1  SampleTime=[1,0]
  dy0 : Outport  Port=15  OutDataTypeStr=double  PortDimensions=1  SampleTime=[1,0]
  dz0 : Outport  Port=16  OutDataTypeStr=double  PortDimensions=1  SampleTime=[1,0]
  delta_Dx : Outport  Port=17  OutDataTypeStr=double  PortDimensions=1  SampleTime=[1,0]
  delta_Dy : Outport  Port=18  OutDataTypeStr=double  PortDimensions=1  SampleTime=[1,0]
  delta_Dz : Outport  Port=19  OutDataTypeStr=double  PortDimensions=1  SampleTime=[1,0]
  rho_a0 : Outport  Port=20  OutDataTypeStr=double  PortDimensions=1  SampleTime=[1,0]
  x : Outport  Port=21  OutDataTypeStr=double  PortDimensions=1  SampleTime=0
  x_dot : Outport  Port=22  OutDataTypeStr=double  PortDimensions=1  SampleTime=0
  y : Outport  Port=23  OutDataTypeStr=double  PortDimensions=1  SampleTime=0
  y_dot : Outport  Port=24  OutDataTypeStr=double  PortDimensions=1  SampleTime=0
  z : Outport  Port=25  OutDataTypeStr=double  PortDimensions=1  SampleTime=0
  z_dot : Outport  Port=26  OutDataTypeStr=double  PortDimensions=1  SampleTime=0
  rho_a1 : Outport  Port=27  OutDataTypeStr=double  PortDimensions=1  SampleTime=[1,0]
  r0_dotdot : Outport  Port=28  OutDataTypeStr=double  PortDimensions=1  SampleTime=0
  omega_z_dot : Outport  Port=29  OutDataTypeStr=double  PortDimensions=1  SampleTime=0
  dx1 : Outport  Port=30  OutDataTypeStr=double  PortDimensions=1  SampleTime=[1,0]
  dy1 : Outport  Port=31  OutDataTypeStr=double  PortDimensions=1  SampleTime=[1,0]
  dz1 : Outport  Port=32  OutDataTypeStr=double  PortDimensions=1  SampleTime=[1,0]
  omega_y_dot : Outport  Port=33  OutDataTypeStr=double  PortDimensions=1  SampleTime=0
  omega_x_dot : Outport  Port=34  OutDataTypeStr=double  PortDimensions=1  SampleTime=0
  i0_dot : Outport  Port=35  OutDataTypeStr=double  PortDimensions=1  SampleTime=0
  ohm0_dot : Outport  Port=36  OutDataTypeStr=double  PortDimensions=1  SampleTime=0
  omega_y : Outport  Port=37  OutDataTypeStr=double  PortDimensions=1  SampleTime=0
  wires:
  DinamicaCinematicaOrbital/6 -> r1/1, [r1]  "r1"
  PerturbacoesOrbitais/4 -> [Vra0]
  DinamicaCinematicaOrbital/8 -> i0/1, [i0]
  DinamicaCinematicaOrbital/12 -> omega_x/1, [omega_x]  "omega_x"
  DinamicaCinematicaOrbital/10 -> theta0_dot/1, [theta0_dot]  "theta0_dot"
  PerturbacoesOrbitais/9 -> rho_a1/1  "rho_a1"
  PerturbacoesOrbitais/7 -> delta_Dz/1, [delta_Dz]
  DinamicaCinematicaOrbital/1 -> x_dotdot/1, [x_dotdot]  "x_dotdot"
  PerturbacoesOrbitais/2 -> [dy0], dy0/1  "dy0"
  DinamicaCinematicaOrbital/9 -> theta0/1, [theta0]
  PerturbacoesOrbitais/6 -> delta_Dy/1, [delta_Dy]
  PerturbacoesOrbitais/1 -> dx0/1, [dx0]  "dx0"
  Model/5 -> z/1, [z]
  Model/4 -> y_dot/1, [y_dot]
  Model/1 -> x/1, [x]
  Model/3 -> y/1, [y]
  PerturbacoesOrbitais/3 -> dz0/1, [dz0]  "dz0"
  DinamicaCinematicaOrbital/7 -> r0_dot/1, [r0_dot]
  PerturbacoesOrbitais/8 -> [rho_a0], rho_a0/1  "rho_a0"
  DinamicaCinematicaOrbital/5 -> h0/1, [h0]
  DinamicaCinematicaOrbital/13 -> omega_z/1, [omega_z]  "omega_z"
  DinamicaCinematicaOrbital/3 -> z_dotdot/1, [z_dotdot]  "z_dotdot"
  DinamicaCinematicaOrbital/2 -> y_dotdot/1, [y_dotdot]  "y_dotdot"
  DinamicaCinematicaOrbital/4 -> r0/1, [r0]
  Model/6 -> z_dot/1, [z_dot]
  DinamicaCinematicaOrbital/11 -> ohm0/1, [ohm0]
  PerturbacoesOrbitais/5 -> delta_Dx/1, [delta_Dx]
  Model/2 -> x_dot/1, [x_dot]
  DinamicaCinematicaOrbital/14 -> r0_dotdot/1, [r0_dotdot]  "r0_dotdot"
  DinamicaCinematicaOrbital/15 -> omega_z_dot/1, [omega_z_dot]  "r0_dotdot"
  PerturbacoesOrbitais/10 -> dx1/1
  PerturbacoesOrbitais/11 -> dy1/1
  PerturbacoesOrbitais/12 -> dz1/1
  DinamicaCinematicaOrbital/16 -> omega_y_dot/1, [omega_y_dot]
  DinamicaCinematicaOrbital/17 -> omega_x_dot/1, [omega_x_dot]
  DinamicaCinematicaOrbital/18 -> i0_dot/1, [i0_dot]
  ? -> [ohm0_dot], ohm0_dot/1
  ? -> [omega_y], omega_y/1
  [dx0] -> DinamicaCinematicaOrbital/1
  [dy0] -> DinamicaCinematicaOrbital/2
  [dz0] -> DinamicaCinematicaOrbital/3
  [x] -> DinamicaCinematicaOrbital/4
  [y] -> ?
  [z] -> ?
  [x_dot] -> ?
  [y_dot] -> ?
  [z_dot] -> ?
  [rho_a0] -> ?
  [Vra0] -> ?
  [delta_Dx] -> ?
  [delta_Dy] -> ?
  [delta_Dz] -> ?
  ux/1 -> ?
  uy/1 -> ?
  uz/1 -> ?
  [z_dot] -> PerturbacoesOrbitais/14
  [y_dot] -> PerturbacoesOrbitais/13
  [x_dot] -> PerturbacoesOrbitais/12
  [z] -> PerturbacoesOrbitais/11
  [y] -> PerturbacoesOrbitais/10
  [r1] -> PerturbacoesOrbitais/9
  [omega_x] -> PerturbacoesOrbitais/8
  [ohm0] -> PerturbacoesOrbitais/7
  [omega_z] -> PerturbacoesOrbitais/6
  [theta0] -> PerturbacoesOrbitais/5
  [i0] -> PerturbacoesOrbitais/4
  [r0_dot] -> PerturbacoesOrbitais/3
  [x] -> PerturbacoesOrbitais/2
  [r0] -> PerturbacoesOrbitais/1
  [x_dotdot] -> Model/1
  [y_dotdot] -> Model/2
  [z_dotdot] -> Model/3
  [theta0_dot] -> Model/4
  [r0_dot] -> Model/5
  [r0] -> Model/6
  [h0] -> Model/7
  Constant1/1 -> Model/8

== system backups/Sensores Atitude ==
  note: Entradas
  note: Sensor de Estrelas
  note: Saídas
  qRelIn : Inport
  Cast To Single : DataTypeConversion  OutDataTypeStr=single  SaturateOnIntegerOverflow=off  RndMeth=Floor
  Constant : Constant  Value=estrelas
  Demux : Demux  Outputs=3
  "Euler -> Quat" : MATLAB Function  TreatAsAtomicUnit=on
  If : If  IfExpression=u1 ~= 0
  Merge : Merge
  Mux1 : Mux  Inputs=3
  "Quat -> Euler" : MATLAB Function  TreatAsAtomicUnit=on
  Sensor ativado : Subsystem  TreatAsAtomicUnit=on
  Sensor desativado : Subsystem  TreatAsAtomicUnit=on
  qRelOut : Outport
  wires:
  Constant/1 -> Cast To Single/1
  Cast To Single/1 -> If/1
  If/1 -> Sensor ativado/Action
  If/2 -> Sensor desativado/Action
  Sensor desativado/1(atitudeOut) -> Merge/2
  Sensor ativado/1(atitudeOut) -> Merge/1
  "Quat -> Euler"/1(phi) -> Mux1/1
  "Quat -> Euler"/3(psi) -> Mux1/3
  "Quat -> Euler"/2(theta) -> Mux1/2
  Merge/1 -> Demux/1
  Demux/3 -> "Euler -> Quat"/3(psi_ref)
  Demux/2 -> "Euler -> Quat"/2(theta_ref)
  Demux/1 -> "Euler -> Quat"/1(phi_ref)
  Mux1/1 -> Sensor desativado/1(atitudeIn), Sensor ativado/1(atitudeIn)
  qRelIn/1 -> [q_rel]
  [q_rel] -> "Quat -> Euler"/1(u)
  [q_rel] -> "Euler -> Quat"/4(q_in)
  "Euler -> Quat"/1(q_ref) -> [q_relOut]
  [q_relOut] -> qRelOut/1

== system backups/Sensores Atitude1 ==
  note: Entradas
  note: Sensor de Estrelas
  note: Saídas
  qRel : Inport
  Cast To Single : DataTypeConversion  OutDataTypeStr=single  SaturateOnIntegerOverflow=off  RndMeth=Floor
  Constant : Constant  Value=estrelas
  Demux : Demux  Outputs=3
  "Euler -> Quatérnions" : MATLAB Function  TreatAsAtomicUnit=on
  If : If  IfExpression=u1 ~= 0
  Merge : Merge
  Mux1 : Mux  Inputs=3
  Sensor ativado : Subsystem  TreatAsAtomicUnit=on
  Sensor desativado : Subsystem  TreatAsAtomicUnit=on
  quat>euler : MATLAB Function  TreatAsAtomicUnit=on
  qRelSen : Outport
  wires:
  Constant/1 -> Cast To Single/1
  Cast To Single/1 -> If/1
  If/1 -> Sensor ativado/Action
  If/2 -> Sensor desativado/Action
  Sensor desativado/1(atitudeSen) -> Merge/2
  Sensor ativado/1(atitudeSen) -> Merge/1
  quat>euler/1(phi) -> Mux1/1
  quat>euler/3(psi) -> Mux1/3
  quat>euler/2(theta) -> Mux1/2
  Merge/1 -> Demux/1
  Demux/3 -> "Euler -> Quatérnions"/3(psi_ref)
  Demux/2 -> "Euler -> Quatérnions"/2(theta_ref)
  Demux/1 -> "Euler -> Quatérnions"/1(phi_ref)
  Mux1/1 -> Sensor ativado/1(atitude), Sensor desativado/1(atitude)
  qRel/1 -> [q_rel]
  [q_rel] -> quat>euler/1(u)
  [q_rel] -> "Euler -> Quatérnions"/4(q_in)
  "Euler -> Quatérnions"/1(q_ref) -> [q_rel_sen]
  [q_rel_sen] -> qRelSen/1

== system backups/Sensores Orbital ==
  note: Entradas
  note: Sensor GNSS/CDGNSS
  note: Saídas
  dinCinOrbIn : Inport
  Cast To Single : DataTypeConversion  OutDataTypeStr=single  SaturateOnIntegerOverflow=off  RndMeth=Floor
  Constant : Constant  Value=cdgps
  If : If  IfExpression=u1 ~= 0
  Merge : Merge
  Sensor ativado : Subsystem  TreatAsAtomicUnit=on
  Sensor desativado : Subsystem  TreatAsAtomicUnit=on
  dinCinOrbOut : Outport
  wires:
  Constant/1 -> Cast To Single/1
  Cast To Single/1 -> If/1
  If/1 -> Sensor ativado/Action
  If/2 -> Sensor desativado/Action
  Sensor desativado/1(dinCinOrbOut) -> Merge/2
  Sensor ativado/1(dinCinOrbOut) -> Merge/1
  dinCinOrbIn/1 -> [dinCinOrb]
  [dinCinOrb] -> Sensor ativado/1(dinCinOrbIn), Sensor desativado/1(dinCinOrbIn)
  Merge/1 -> [dinCinOrbSen]
  [dinCinOrbSen] -> dinCinOrbOut/1

== system backups/Sensores Orbital1 ==
  note: Entradas
  note: Sensor GNSS/CDGNSS
  note: Saídas
  dinCinOrb : Inport
  Cast To Single : DataTypeConversion  OutDataTypeStr=single  SaturateOnIntegerOverflow=off  RndMeth=Floor
  Constant : Constant  Value=cdgps
  If : If  IfExpression=u1 ~= 0
  Merge : Merge
  Sensor ativado : Subsystem  TreatAsAtomicUnit=on
  Sensor desativado : Subsystem  TreatAsAtomicUnit=on
  dinCinOrbSen : Outport
  wires:
  Constant/1 -> Cast To Single/1
  Cast To Single/1 -> If/1
  If/1 -> Sensor ativado/Action
  If/2 -> Sensor desativado/Action
  Sensor desativado/1(Out1) -> Merge/2
  Sensor ativado/1(Out1) -> Merge/1
  dinCinOrb/1 -> [dinCinOrb]
  [dinCinOrb] -> Sensor ativado/1(dinCinOrb), Sensor desativado/1(dinCinOrb)
  Merge/1 -> [dinCinOrbSen]
  [dinCinOrbSen] -> dinCinOrbSen/1

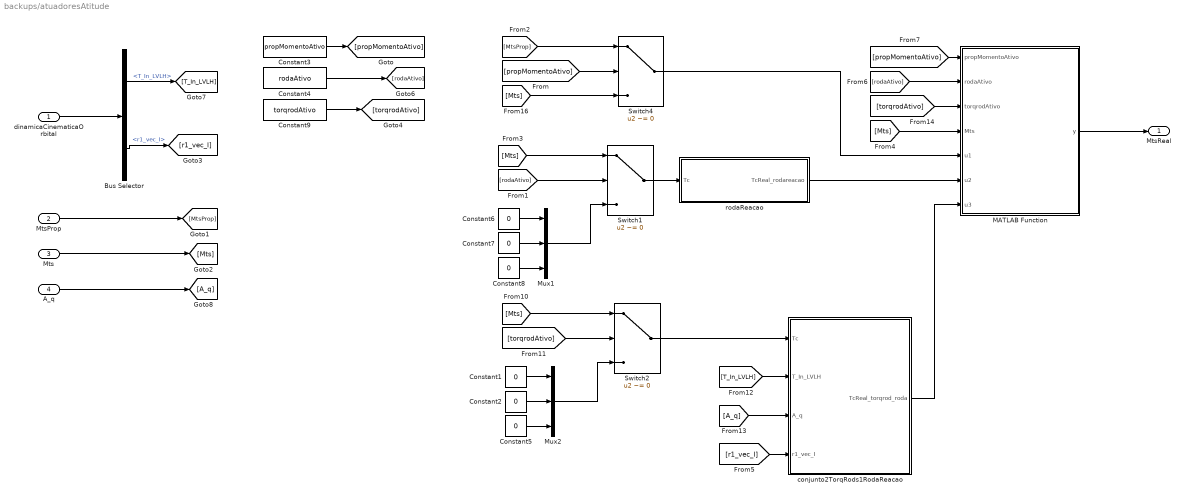
== system backups/atuadoresAtitude ==
  dinamicaCinematicaOrbital : Inport
  MtsProp : Inport  Port=2
  Mts : Inport  Port=3
  A_q : Inport  Port=4
  Bus Selector : BusSelector  OutputSignals=T_In_LVLH,r1_vec_I
  Constant{1..2,5..8} (6 alike) : Constant  Value=0  SampleTime=-1
  Constant3 : Constant  Value=propMomentoAtivo  SampleTime=-1
  Constant4 : Constant  Value=rodaAtivo  SampleTime=-1
  Constant9 : Constant  Value=torqrodAtivo  SampleTime=-1
  MATLAB Function : MATLAB Function  TreatAsAtomicUnit=on
  Mux1 : Mux  Inputs=3
  Mux2 : Mux  Inputs=3
  Switch1 : Switch  Criteria=u2 ~= 0  SaturateOnIntegerOverflow=off  InputSameDT=off
  Switch2 : Switch  Criteria=u2 ~= 0  SaturateOnIntegerOverflow=off  InputSameDT=off
  Switch4 : Switch  Criteria=u2 ~= 0  SaturateOnIntegerOverflow=off  InputSameDT=off
  conjunto2TorqRods1RodaReacao : Subsystem
  rodaReacao : Subsystem
  MtsReal : Outport
  wires:
  Constant4/1 -> [rodaAtivo]
  Constant3/1 -> [propMomentoAtivo]
  Mts/1 -> [Mts]
  dinamicaCinematicaOrbital/1 -> Bus Selector/1
  [propMomentoAtivo] -> Switch4/2
  [rodaAtivo] -> Switch1/2
  [Mts] -> Switch1/1
  Constant8/1 -> Mux1/3
  Constant7/1 -> Mux1/2
  Mux1/1 -> Switch1/3
  Constant6/1 -> Mux1/1
  Switch1/1 -> rodaReacao/1(Tc)
  MtsProp/1 -> [MtsProp]
  [MtsProp] -> Switch4/1
  rodaReacao/1(TcReal_rodareacao) -> MATLAB Function/6(u2)
  Switch4/1 -> MATLAB Function/5(u1)
  [rodaAtivo] -> MATLAB Function/2(rodaAtivo)
  [propMomentoAtivo] -> MATLAB Function/1(propMomentoAtivo)
  A_q/1 -> [A_q]
  Constant9/1 -> [torqrodAtivo]
  [torqrodAtivo] -> MATLAB Function/3(torqrodAtivo)
  MATLAB Function/1(y) -> MtsReal/1
  Bus Selector/1 -> [T_In_LVLH]  "<T_In_LVLH>"
  [Mts] -> Switch4/3
  [Mts] -> MATLAB Function/4(Mts)
  Bus Selector/2 -> [r1_vec_I]  "<r1_vec_I>"
  conjunto2TorqRods1RodaReacao/1(TcReal_torqrod_roda) -> MATLAB Function/7(u3)
  [T_In_LVLH] -> conjunto2TorqRods1RodaReacao/2(T_In_LVLH)
  Constant1/1 -> Mux2/1
  [r1_vec_I] -> conjunto2TorqRods1RodaReacao/4(r1_vec_I)
  [torqrodAtivo] -> Switch2/2
  Constant2/1 -> Mux2/2
  Switch2/1 -> conjunto2TorqRods1RodaReacao/1(Tc)
  [Mts] -> Switch2/1
  Mux2/1 -> Switch2/3
  [A_q] -> conjunto2TorqRods1RodaReacao/3(A_q)
  Constant5/1 -> Mux2/3

== system backups/atuadoresOrbital ==
  A_q : Inport
  controleOrbital : Inport  Port=2
  Mts : Inport  Port=3
  AtuadorNaoLinear : ModelReference  ModelNameDialog=AtuadorNaoLinear  ModelReferenceVersion=3.54
  Constant{,1..2,6..8} (6 alike) : Constant  Value=0  SampleTime=-1
  Constant3 : Constant  Value=propMomentoAtivo  SampleTime=-1
  Constant5 : Constant  Value=propForcaAtivo  SampleTime=-1
  Mux : Mux  Inputs=3
  Mux1 : Mux  Inputs=3
  Switch{1..4} (4 alike) : Switch  Criteria=u2 ~= 0  SaturateOnIntegerOverflow=off  InputSameDT=off
  acelControle : Outport
  MtsProp : Outport  Port=2
  wires:
  Constant7/1 -> Mux1/2
  A_q/1 -> [A_q]
  [propForcaAtivo] -> Switch2/2
  Mux/1 -> Switch4/3
  [propMomentoAtivo] -> Switch1/2
  Constant/1 -> Mux/1
  [controleOrbital] -> Switch3/3
  Mux1/1 -> Switch2/3
  [propMomentoAtivo] -> Switch4/2
  [A_q] -> AtuadorNaoLinear/1
  [controleOrbital] -> Switch2/1
  [acelControleProp] -> Switch3/1
  AtuadorNaoLinear/1 -> [acelControleProp]
  [Mts] -> Switch1/3
  controleOrbital/1 -> [controleOrbital]
  [Mts] -> Switch4/1
  AtuadorNaoLinear/2 -> [torquesProp]
  Switch4/1 -> ?
  Switch2/1 -> AtuadorNaoLinear/2
  Constant1/1 -> Mux/2
  Mts/1 -> [Mts]
  [propForcaAtivo] -> Switch3/2
  Constant3/1 -> [propMomentoAtivo]
  Constant8/1 -> Mux1/3
  Constant6/1 -> Mux1/1
  [torquesProp] -> Switch1/1
  Constant5/1 -> [propForcaAtivo]
  Constant2/1 -> Mux/3
  Switch1/1 -> MtsProp/1
  Switch3/1 -> acelControle/1

== system backups/atuadoresOrbital1 ==
  note: A_q, controleOrbital e Mts possuiam um unit delay block
  A_q : Inport
  controleOrbital : Inport  Port=2
  Mts : Inport  Port=3
  AtuadorNaoLinear : ModelReference  ModelNameDialog=AtuadorNaoLinear  ModelReferenceVersion=3.54
  Constant10 : Constant  Value=[0 0 0]
  Constant3 : Constant  Value=propMomentoAtivo  SampleTime=-1
  Constant4 : Constant  Value=m1  SampleTime=-1
  Constant5 : Constant  Value=propForcaAtivo  SampleTime=-1
  Constant6 : Constant  Value=[0 0 0]
  Constant9 : Constant  Value=m1  SampleTime=-1
  Mux2 : Mux  Inputs=3
  Mux3 : Mux  Inputs=3
  Switch{1..4} (4 alike) : Switch  Criteria=u2 ~= 0  SaturateOnIntegerOverflow=off  InputSameDT=off
  Unit Delay1 : UnitDelay  SampleTime=-1  HasFrameUpgradeWarning=on
  Unit Delay2 : UnitDelay  SampleTime=-1  HasFrameUpgradeWarning=on
  Unit Delay3 : UnitDelay  SampleTime=-1  HasFrameUpgradeWarning=on
  acelSistLVLHSeg1 : MATLAB Function  TreatAsAtomicUnit=on
  forçasSistCorpoSeg : MATLAB Function  TreatAsAtomicUnit=on
  acelControle : Outport
  MtsProp : Outport  Port=2
  wires:
  A_q/1 -> Unit Delay1/1
  [propForcaAtivo] -> Switch2/2
  [propMomentoAtivo] -> Switch1/2
  [controleOrbital] -> Switch3/3
  [propMomentoAtivo] -> Switch4/2
  [controleOrbital] -> Switch2/1
  [acelControleProp] -> Switch3/1
  [Mts] -> Switch1/3
  controleOrbital/1 -> Unit Delay2/1
  [Mts] -> Switch4/1
  AtuadorNaoLinear/2 -> [torquesProp]
  Mts/1 -> Unit Delay3/1
  [propForcaAtivo] -> Switch3/2
  Constant3/1 -> [propMomentoAtivo]
  [torquesProp] -> Switch1/1
  Constant5/1 -> [propForcaAtivo]
  Switch1/1 -> MtsProp/1
  Switch3/1 -> acelControle/1
  Switch4/1 -> AtuadorNaoLinear/2
  AtuadorNaoLinear/1 -> acelSistLVLHSeg1/3(F_b)
  acelSistLVLHSeg1/1(acelx) -> Mux3/1
  acelSistLVLHSeg1/3(acelz) -> Mux3/3
  acelSistLVLHSeg1/2(acely) -> Mux3/2
  Constant4/1 -> acelSistLVLHSeg1/2(m1)
  Mux3/1 -> [acelControleProp]  "OutReal"
  [A_q] -> acelSistLVLHSeg1/1(A_q)
  forçasSistCorpoSeg/3(Fz_b) -> Mux2/3
  Constant9/1 -> forçasSistCorpoSeg/2(m1)
  Mux2/1 -> AtuadorNaoLinear/1
  forçasSistCorpoSeg/1(Fx_b) -> Mux2/1
  [A_q] -> forçasSistCorpoSeg/1(A_q)
  forçasSistCorpoSeg/2(Fy_b) -> Mux2/2
  Unit Delay1/1 -> [A_q]
  Unit Delay2/1 -> [controleOrbital]
  Unit Delay3/1 -> [Mts]
  Switch2/1 -> forçasSistCorpoSeg/3(controleOrbital)
  Constant10/1 -> Switch2/3
  Constant6/1 -> Switch4/3

== system backups/controleOrbital ==
  note: Planta
  note: Saídas
  note: Entradas
  errosOrbital : Inport
  Add : Sum  Inputs=+++
  Add1 : Sum  Inputs=+++
  Add2 : Sum  Inputs=+++
  Bus Selector : BusSelector  OutputSignals=erro_x,erro_x_dot,erro_y,erro_y_dot,erro_z,erro_z_dot
  Integrator : Integrator
  Integrator1 : Integrator
  Integrator2 : Integrator
  Mux : Mux  Inputs=3
  OrbKd_x1 : Gain  Gain=OrbKd_x
  OrbKd_y1 : Gain  Gain=OrbKd_y
  OrbKd_z1 : Gain  Gain=OrbKd_z
  OrbKi_x1 : Gain  Gain=OrbKi_x
  OrbKi_y1 : Gain  Gain=OrbKi_y
  OrbKi_z1 : Gain  Gain=OrbKi_z
  OrbKp_x1 : Gain  Gain=OrbKp_x
  OrbKp_y1 : Gain  Gain=OrbKp_y
  OrbKp_z1 : Gain  Gain=OrbKp_z
  Scope : Scope
  controleOrbital : Outport
  wires:
  [erro_y] -> OrbKp_y1/1, Integrator1/1
  Integrator2/1 -> OrbKi_z1/1
  [ux] -> Mux/1  "ux"
  Mux/1 -> controleOrbital/1, Scope/1
  OrbKi_z1/1 -> Add2/2
  [uz] -> Mux/3  "uz"
  Bus Selector/1 -> [erro_x]  "<erro_x>"
  Integrator1/1 -> OrbKi_y1/1
  [erro_x_dot] -> OrbKd_x1/1
  Bus Selector/6 -> [erro_z_dot]  "<erro_z_dot>"
  Bus Selector/3 -> [erro_y]  "<erro_y>"
  OrbKp_z1/1 -> Add2/1
  errosOrbital/1 -> Bus Selector/1
  Bus Selector/4 -> [erro_y_dot]  "<erro_y_dot>"
  [erro_z_dot] -> OrbKd_z1/1
  OrbKd_z1/1 -> Add2/3
  [erro_z] -> OrbKp_z1/1, Integrator2/1
  OrbKd_y1/1 -> Add1/3
  Add2/1 -> [uz]
  [uy] -> Mux/2  "uy"
  [erro_y_dot] -> OrbKd_y1/1
  Add/1 -> [ux]
  Integrator/1 -> OrbKi_x1/1
  OrbKp_y1/1 -> Add1/1
  OrbKi_y1/1 -> Add1/2
  [erro_x] -> OrbKp_x1/1, Integrator/1
  OrbKd_x1/1 -> Add/3
  OrbKp_x1/1 -> Add/1
  Add1/1 -> [uy]
  Bus Selector/5 -> [erro_z]  "<erro_z>"
  OrbKi_x1/1 -> Add/2
  Bus Selector/2 -> [erro_x_dot]  "<erro_x_dot>"

== system backups/dinamicaCinematicaAtitude1 ==
  note: Planta
  note: Saídas
  note: Entradas
  dinamicaCinematicaOrbital : Inport
  Mts : Inport  Port=2
  Bus Creator : BusCreator  Inputs=3
  Bus Selector : BusSelector  OutputSignals=omega_x,omega_y,omega_z,omega_x_dot,omega_y_dot,omega_z_dot
  DinamicaCinematicaAtitude : ModelReference  ModelNameDialog=DinamicaCinematicaControleAtitude  ModelReferenceVersion=3.14
  MATLAB Function : MATLAB Function  TreatAsAtomicUnit=on
  Vector Concatenate : Concatenate  NumInputs=3  Mode=Multidimensional array
  Vector Concatenate1 : Concatenate  NumInputs=3  Mode=Multidimensional array
  euler : Outport
  q_rel : Outport  Port=2
  A_q : Outport  Port=3
  omega_rel : Outport  Port=4
  wires:
  DinamicaCinematicaAtitude/1 -> [q_rel]
  DinamicaCinematicaAtitude/2 -> [A_q]
  [q_rel] -> q_rel/1
  [A_q] -> A_q/1
  dinamicaCinematicaOrbital/1 -> Bus Selector/1
  [omega_i] -> DinamicaCinematicaAtitude/2
  [omega_i_dot] -> DinamicaCinematicaAtitude/3
  [Mts] -> DinamicaCinematicaAtitude/1
  Bus Selector/1 -> Vector Concatenate1/1  "<omega_x>"
  Bus Selector/3 -> Vector Concatenate1/3  "<omega_z>"
  Bus Selector/2 -> Vector Concatenate1/2  "<omega_y>"
  Vector Concatenate1/1 -> [omega_i]
  Bus Selector/4 -> Vector Concatenate/1  "<omega_x_dot>"
  Bus Selector/5 -> Vector Concatenate/2  "<omega_y_dot>"
  Bus Selector/6 -> Vector Concatenate/3  "<omega_z_dot>"
  Vector Concatenate/1 -> [omega_i_dot]
  DinamicaCinematicaAtitude/3 -> [omega_rel]
  [omega_rel] -> omega_rel/1
  Mts/1 -> [Mts]
  [q_rel] -> MATLAB Function/1(u)
  MATLAB Function/1(phi) -> Bus Creator/1
  MATLAB Function/2(theta) -> Bus Creator/2
  MATLAB Function/3(psi) -> Bus Creator/3
  Bus Creator/1 -> euler/1

== system backups/errosAngAtitude1 ==
  note: Planta
  note: Saídas
  note: Entradas
  q_ref : Inport
  q_rel : Inport  Port=2
  MATLAB Function4 : MATLAB Function  TreatAsAtomicUnit=on
  q_erro : Outport
  wires:
  [q_ref] -> MATLAB Function4/1(q_d)
  [q_rel] -> MATLAB Function4/2(q)
  MATLAB Function4/1(q_error) -> [q_erro]  "q_erro"
  [q_erro] -> q_erro/1
  q_rel/1 -> [q_rel]  "q_rel"
  q_ref/1 -> [q_ref]  "eulerRef"

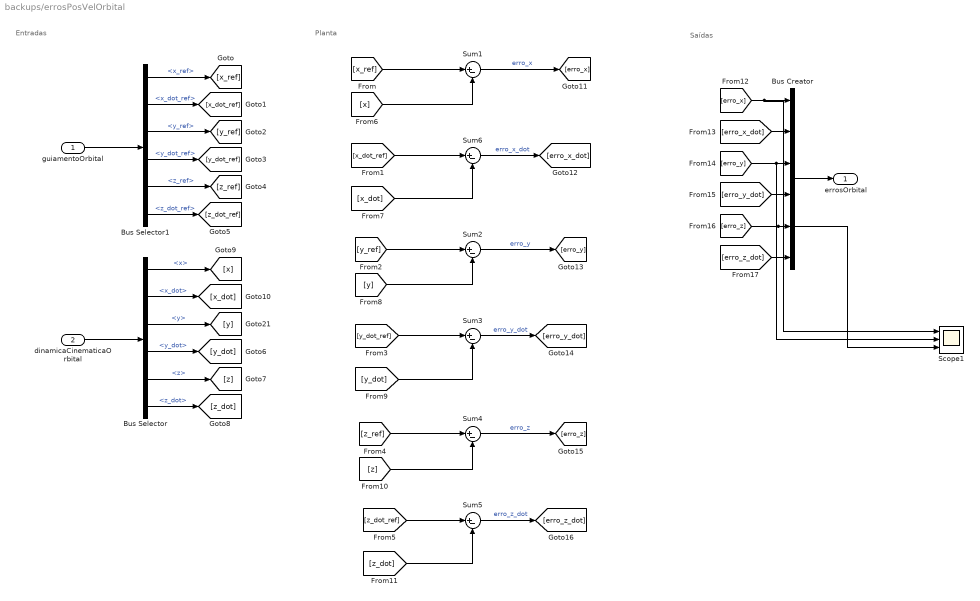
== system backups/errosPosVelOrbital ==
  note: Saídas
  note: Planta
  note: Entradas
  guiamentoOrbital : Inport
  dinamicaCinematicaOrbital : Inport  Port=2
  Bus Creator : BusCreator  Inputs=6
  Bus Selector : BusSelector  OutputSignals=x,x_dot,y,y_dot,z,z_dot
  Bus Selector1 : BusSelector  OutputSignals=x_ref,x_dot_ref,y_ref,y_dot_ref,z_ref,z_dot_ref
  Scope1 : Scope  NumInputPorts=3
  Sum{1..6} (6 alike) : Sum  Inputs=|+-
  errosOrbital : Outport
  wires:
  [x] -> Sum1/2
  [x_dot] -> Sum6/2
  [x_dot_ref] -> Sum6/1
  [x_ref] -> Sum1/1
  Sum6/1 -> [erro_x_dot]  "erro_x_dot"
  Sum1/1 -> [erro_x]  "erro_x"
  Sum3/1 -> [erro_y_dot]  "erro_y_dot"
  Sum2/1 -> [erro_y]  "erro_y"
  [y] -> Sum2/2
  [y_dot] -> Sum3/2
  [y_ref] -> Sum2/1
  [y_dot_ref] -> Sum3/1
  Sum5/1 -> [erro_z_dot]  "erro_z_dot"
  Sum4/1 -> [erro_z]  "erro_z"
  [z_dot] -> Sum5/2
  [z_dot_ref] -> Sum5/1
  [z] -> Sum4/2
  [z_ref] -> Sum4/1
  Bus Selector1/4 -> [y_dot_ref]  "<y_dot_ref>"
  Bus Selector1/2 -> [x_dot_ref]  "<x_dot_ref>"
  guiamentoOrbital/1 -> Bus Selector1/1
  Bus Selector1/6 -> [z_dot_ref]  "<z_dot_ref>"
  Bus Selector1/3 -> [y_ref]  "<y_ref>"
  Bus Selector1/1 -> [x_ref]  "<x_ref>"
  Bus Selector1/5 -> [z_ref]  "<z_ref>"
  Bus Selector/1 -> [x]  "<x>"
  Bus Selector/4 -> [y_dot]  "<y_dot>"
  Bus Selector/3 -> [y]  "<y>"
  Bus Selector/6 -> [z_dot]  "<z_dot>"
  Bus Selector/5 -> [z]  "<z>"
  Bus Selector/2 -> [x_dot]  "<x_dot>"
  dinamicaCinematicaOrbital/1 -> Bus Selector/1
  [erro_x] -> Scope1/1, Bus Creator/1
  [erro_x_dot] -> Bus Creator/2
  [erro_y] -> Scope1/2, Bus Creator/3
  [erro_y_dot] -> Bus Creator/4
  [erro_z] -> Scope1/3, Bus Creator/5
  [erro_z_dot] -> Bus Creator/6
  Bus Creator/1 -> errosOrbital/1

== system backups/Atuadores Orbital/Consumo ==
  Input : Inport
  Abs1 : Abs  SaturateOnIntegerOverflow=off
  Abs2 : Abs  SaturateOnIntegerOverflow=off
  Abs3 : Abs  SaturateOnIntegerOverflow=off
  Add3 : Sum  Inputs=+++
  Demux : Demux  Outputs=3
  Integrator1 : Integrator
  Integrator2 : Integrator
  Integrator3 : Integrator
  Out1 : Outport  VectorParamsAs1DForOutWhenUnconnected=off
  wires:
  Demux/1 -> Abs3/1  "Fx"
  Integrator2/1 -> Add3/2
  Demux/2 -> Abs1/1  "Fy"
  Demux/3 -> Abs2/1  "Fz"
  Integrator3/1 -> Add3/3
  Add3/1 -> Out1/1
  Abs3/1 -> Integrator1/1
  Abs1/1 -> Integrator2/1
  Abs2/1 -> Integrator3/1
  Integrator1/1 -> Add3/1
  Input/1 -> Demux/1

== system backups/Atuadores Orbital/Propulsor ativado ==
  note: Entradas
  note: Propulsores
  note: Saídas
  F_b : Inport
  Tc : Inport  Port=2
  Action Port : ActionPort  ActionPortLabel=if(u1 > 0)
  AtuadorNaoLinear : ModelReference  ModelNameDialog=AtuadorNaoLinear  ModelReferenceVersion=3.54
  forcasPropulsor : Outport
  torquesProp : Outport  Port=2
  wires:
  AtuadorNaoLinear/2 -> [torquesProp]
  AtuadorNaoLinear/1 -> [forcasProp]
  Tc/1 -> [Tc]
  [Tc] -> AtuadorNaoLinear/2
  F_b/1 -> [F_b]
  [F_b] -> AtuadorNaoLinear/1
  [forcasProp] -> forcasPropulsor/1
  [torquesProp] -> torquesProp/1

== system backups/Atuadores Orbital/Propulsor não ativado ==
  F_b : Inport
  Mts : Inport  Port=2
  Action Port : ActionPort  ActionPortLabel=else
  F_b_Out : Outport
  MtsOut : Outport  Port=2
  wires:
  F_b/1 -> F_b_Out/1
  Mts/1 -> MtsOut/1

== system backups/Atuadores Orbital1/Consumo ==
  Input : Inport
  Abs1 : Abs  SaturateOnIntegerOverflow=off
  Abs2 : Abs  SaturateOnIntegerOverflow=off
  Abs3 : Abs  SaturateOnIntegerOverflow=off
  Add3 : Sum  Inputs=+++
  Demux : Demux  Outputs=3
  Integrator1 : Integrator
  Integrator2 : Integrator
  Integrator3 : Integrator
  Out1 : Outport  VectorParamsAs1DForOutWhenUnconnected=off
  wires:
  Demux/1 -> Abs3/1  "Fx"
  Integrator2/1 -> Add3/2
  Demux/2 -> Abs1/1  "Fy"
  Demux/3 -> Abs2/1  "Fz"
  Integrator3/1 -> Add3/3
  Add3/1 -> Out1/1
  Abs3/1 -> Integrator1/1
  Abs1/1 -> Integrator2/1
  Abs2/1 -> Integrator3/1
  Integrator1/1 -> Add3/1
  Input/1 -> Demux/1

== system backups/Atuadores Orbital1/Propulsor ativado ==
  note: Entradas
  note: Propulsores
  note: Saídas
  F_b : Inport
  Tc : Inport  Port=2
  Action Port : ActionPort
  AtuadorNaoLinear : ModelReference  ModelNameDialog=AtuadorNaoLinear  ModelReferenceVersion=3.54
  Cast To Single2 : DataTypeConversion  OutDataTypeStr=single  SaturateOnIntegerOverflow=off  RndMeth=Floor
  Constant1 : Constant  Value=rodaAtivo  SampleTime=-1
  Constant2 : Constant  Value=torqrodAtivo  SampleTime=-1
  If Action Subsystem : Subsystem  TreatAsAtomicUnit=on
  If Action Subsystem1 : Subsystem  TreatAsAtomicUnit=on
  If2 : If
  Logical Operator1 : Logic  Operator=OR  AllPortsSameDT=off  OutDataTypeStr=boolean
  Merge2 : Merge
  forcasPropulsor : Outport
  torquesProp : Outport  Port=2
  wires:
  AtuadorNaoLinear/2 -> [torquesProp]
  AtuadorNaoLinear/1 -> [forcasProp]
  Tc/1 -> [Tc]
  Merge2/1 -> AtuadorNaoLinear/2
  F_b/1 -> [F_b]
  [F_b] -> AtuadorNaoLinear/1
  [forcasProp] -> forcasPropulsor/1
  [torquesProp] -> torquesProp/1
  Constant1/1 -> Logical Operator1/1
  Cast To Single2/1 -> If2/1
  Logical Operator1/1 -> Cast To Single2/1
  Constant2/1 -> Logical Operator1/2
  If2/1 -> If Action Subsystem/Action
  If2/2 -> If Action Subsystem1/Action
  [Tc] -> If Action Subsystem1/1(In1), If Action Subsystem/1(In1)
  If Action Subsystem1/1(Out1) -> Merge2/2
  If Action Subsystem/1(Out1) -> Merge2/1

== system backups/Atuadores Orbital1/Propulsor não ativado ==
  F_b : Inport
  Mts : Inport  Port=2
  Action Port : ActionPort
  F_b_Out : Outport
  MtsOut : Outport  Port=2
  wires:
  F_b/1 -> F_b_Out/1
  Mts/1 -> MtsOut/1
